simulink model "quad_drag_ssmethod"  (R2015b)
settings: Solver=VariableStepAuto  StartTime=0.0  StopTime=10  RelTol=1e-3
settings Model: Creator=bsb  LastModifiedBy=aschnieders22
settings ConfigComp: CovModelRefEnable=Off
settings ConfigurationSet: Description=Simscape Multibody

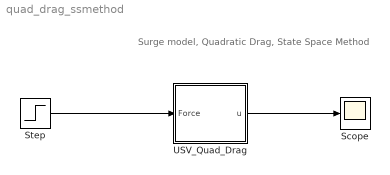
== system quad_drag_ssmethod ==
  note: Surge model, Quadratic Drag, State Space Method
  Scope : Scope
  Step : Step  After=21  SampleTime=0
  USV_Quad_Drag : Subsystem
  wires:
  Step/1 -> USV_Quad_Drag/1(Force)
  USV_Quad_Drag/1(u) -> Scope/1

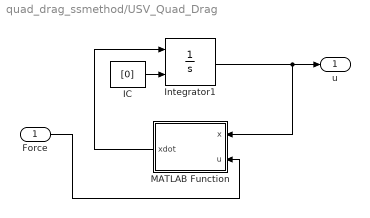
== system quad_drag_ssmethod/USV_Quad_Drag ==
  Force : Inport
  IC : Constant  Value=[0]
  Integrator1 : Integrator  InitialConditionSource=external
  MATLAB Function : MATLAB Function  TreatAsAtomicUnit=on
  u : Outport
  wires:
  IC/1 -> Integrator1/2
  MATLAB Function/1(xdot) -> Integrator1/1
  Integrator1/1 -> u/1, MATLAB Function/1(x)
  Force/1 -> MATLAB Function/2(u)

== matlab function quad_drag_ssmethod/USV_Quad_Drag/MATLAB Function ==
  data: x input; u input; xdot output
function xdot = fcn(x,u)
%#codegen

% x - state of the system.  surge velocity.
% u - input. thrust force
% Model parameters
m = 28.0;   % Mass [kg]
d = 16.9;  % Quadratic drag coefficient [N/(m/s)^2]

xdot = 1/m*(-d*abs(x)*x+u);
